simulink subsystem "block_admittance_controller_transl"  (R2021b)
settings: Solver=VariableStepAuto  StartTime=0.0  StopTime=10.0  RelTol=1e-3
undefined symbols (not defined in the file): dp_cd0, Kd, Kp, Md, p_cd0
settings Model: Creator=Martin  LastModifiedBy=Martin

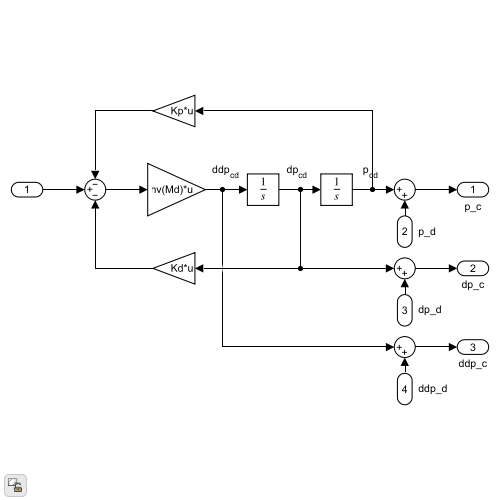
[thumbnail: Simulink's stored preview of the top-level diagram]
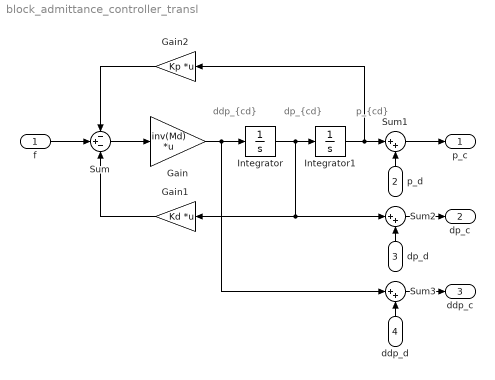
== system block_admittance_controller_transl ==
  note: p_{cd}
  note: dp_{cd}
  note: ddp_{cd}
  f : Inport  PortDimensions=[3 1]
  p_d : Inport  Port=2  PortDimensions=[3 1]
  dp_d : Inport  Port=3  PortDimensions=[3 1]
  ddp_d : Inport  Port=4  PortDimensions=[3 1]
  Gain : Gain  Gain=inv(Md)  Multiplication=Matrix(K*u)
  Gain1 : Gain  Gain=Kd  Multiplication=Matrix(K*u)
  Gain2 : Gain  Gain=Kp  Multiplication=Matrix(K*u)
  Integrator : Integrator  InitialCondition=dp_cd0
  Integrator1 : Integrator  InitialCondition=p_cd0
  Sum : Sum  Inputs=-+-
  Sum1 : Sum  Inputs=|++
  Sum2 : Sum  Inputs=|++
  Sum3 : Sum  Inputs=|++
  p_c : Outport
  dp_c : Outport  Port=2
  ddp_c : Outport  Port=3
  wires:
  Sum2/1 -> dp_c/1
  Sum3/1 -> ddp_c/1
  Integrator/1 -> Integrator1/1, Sum2/1, Gain1/1
  Integrator1/1 -> Gain2/1, Sum1/1
  dp_d/1 -> Sum2/2
  Gain/1 -> Integrator/1, Sum3/1
  ddp_d/1 -> Sum3/2
  Sum1/1 -> p_c/1
  f/1 -> Sum/2
  p_d/1 -> Sum1/2
  Sum/1 -> Gain/1
  Gain2/1 -> Sum/1
  Gain1/1 -> Sum/3
